simulink model "OMAP"  (R2018b)
settings: Solver=FixedStepDiscrete  StartTime=0.0  StopTime=10.0  FixedStep=0.01  RelTol=1e-3
values from neighbouring files (symbols this model uses):
  Clb_ICADirect_LaneDisp_StateFive = Simulink.Parameter    [omap_ver_442.m]
  Clb_ICADirect_LaneDisp_StateFour = Simulink.Parameter    [omap_ver_442.m]
  Clb_ICADirect_LaneDisp_StateOne = Simulink.Parameter    [omap_ver_442.m]
  Clb_ICADirect_LaneDisp_StateThree = Simulink.Parameter    [omap_ver_442.m]
  Clb_ICADirect_LaneDisp_StateTwo = Simulink.Parameter    [omap_ver_442.m]
  Clb_ICADirect_LaneDisp_StateZero = Simulink.Parameter    [omap_ver_442.m]
  Clb_ICADirect_LaneDispSW = Simulink.Parameter    [omap_ver_442.m]
  Clb_ICADirect_TrnLghtsCom_Switch = Simulink.Parameter    [omap_ver_442.m]
  Clb_ICADirect_TrnLghtsCom_Value = Simulink.Parameter    [omap_ver_442.m]
  Clb_ICADirect_TrnLghtsCrtl_Inhb = Simulink.Parameter    [omap_ver_442.m]
  OMAP_ACCAEB_EMSESC_Decel = Simulink.Parameter    [omap_ver_442.m]
  OMAP_ACCFCW_IC_Decel = Simulink.Parameter    [omap_ver_442.m]
  OMAP_clb_ACC_RVVReqType = Simulink.Parameter    [omap_ver_442.m]
  OMAP_clb_ACC_RVVReqType_Switch = Simulink.Parameter    [omap_ver_442.m]
  OMAP_clb_ACCHeadwayDisplay = Simulink.Parameter    [omap_ver_442.m]
  OMAP_clb_ACCHeadwayDisplay_Switch = Simulink.Parameter    [omap_ver_442.m]
  OMAP_clb_ACCHeadwayIcon = Simulink.Parameter    [omap_ver_442.m]
  OMAP_clb_ACCHeadwayIcon_Switch = Simulink.Parameter    [omap_ver_442.m]
  OMAP_clb_ACCMessagePrompt = Simulink.Parameter    [omap_ver_442.m]
  OMAP_clb_ACCMessagePrompt_Switch = Simulink.Parameter    [omap_ver_442.m]
  OMAP_clb_ACCRequestEPB = Simulink.Parameter    [omap_ver_442.m]
  OMAP_clb_ACCRequestEPB_Switch = Simulink.Parameter    [omap_ver_442.m]
  OMAP_clb_ACCSetSpeed = Simulink.Parameter    [omap_ver_442.m]
  OMAP_clb_ACCSetSpeed_Switch = Simulink.Parameter    [omap_ver_442.m]
  OMAP_clb_ACCSetSpeedDis = Simulink.Parameter    [omap_ver_442.m]
  OMAP_clb_ACCSetSpeedDis_Switch = Simulink.Parameter    [omap_ver_442.m]
  OMAP_clb_ACCState = Simulink.Parameter    [omap_ver_442.m]
  OMAP_clb_ACCState_Switch = Simulink.Parameter    [omap_ver_442.m]
  OMAP_clb_ACCStatusIconDis = Simulink.Parameter    [omap_ver_442.m]
  OMAP_clb_ACCStatusIconDis_Switch = Simulink.Parameter    [omap_ver_442.m]
  OMAP_clb_ACCTorqueReq = Simulink.Parameter    [omap_ver_442.m]
  OMAP_clb_ACCTorqueReq_Switch = Simulink.Parameter    [omap_ver_442.m]
  OMAP_clb_ADAS_State = Simulink.Parameter    [omap_ver_442.m]
  OMAP_clb_ADAS_State_Switch = Simulink.Parameter    [omap_ver_442.m]
  OMAP_clb_AEBAlertReq = Simulink.Parameter    [omap_ver_442.m]
  OMAP_clb_AEBAlertReq_Switch = Simulink.Parameter    [omap_ver_442.m]
  OMAP_clb_AEBBrakingProg = Simulink.Parameter    [omap_ver_442.m]
  OMAP_clb_AEBBrakingProg_Switch = Simulink.Parameter    [omap_ver_442.m]
  OMAP_clb_AEBFaultStatus = Simulink.Parameter    [omap_ver_442.m]
  OMAP_clb_AEBFaultStatus_Switch = Simulink.Parameter    [omap_ver_442.m]
  OMAP_clb_AEBMassageDisp = Simulink.Parameter    [omap_ver_442.m]
  OMAP_clb_AEBMassageDisp_Switch = Simulink.Parameter    [omap_ver_442.m]
  OMAP_clb_AEBState = Simulink.Parameter    [omap_ver_442.m]
  OMAP_clb_AEBState_Switch = Simulink.Parameter    [omap_ver_442.m]
  OMAP_clb_AEBSwitchStatus = Simulink.Parameter    [omap_ver_442.m]
  OMAP_clb_AEBSwitchStatus_Switch = Simulink.Parameter    [omap_ver_442.m]
  OMAP_clb_BrakeRequest = Simulink.Parameter    [omap_ver_442.m]
  OMAP_clb_BrakeRequest_Switch = Simulink.Parameter    [omap_ver_442.m]
  OMAP_clb_DecelerationSet = Simulink.Parameter    [omap_ver_442.m]
  OMAP_clb_DecelerationSet_Switch = Simulink.Parameter    [omap_ver_442.m]
  OMAP_clb_DecelerationType = Simulink.Parameter    [omap_ver_442.m]
  OMAP_clb_DecelerationType_Switch = Simulink.Parameter    [omap_ver_442.m]
  OMAP_clb_DeclControlReq = Simulink.Parameter    [omap_ver_442.m]
  OMAP_clb_DeclControlReq_Switch = Simulink.Parameter    [omap_ver_442.m]
  OMAP_clb_DownorUpGearMinTime = Simulink.Parameter    [omap_ver_442.m]
  OMAP_clb_DownorUpGearMinTime_Switch = Simulink.Parameter    [omap_ver_442.m]
  OMAP_clb_ELKPopupMessage = Simulink.Parameter    [omap_ver_442.m]
  OMAP_clb_ELKPopupMessage_Switch = Simulink.Parameter    [omap_ver_442.m]
  OMAP_clb_ELKSts = Simulink.Parameter    [omap_ver_442.m]
  OMAP_clb_ELKSts_Switch = Simulink.Parameter    [omap_ver_442.m]
  OMAP_clb_ESAFaultSt = Simulink.Parameter    [omap_ver_442.m]
  OMAP_clb_ESAFaultSt_Switch = Simulink.Parameter    [omap_ver_442.m]
  OMAP_clb_ESARequest = Simulink.Parameter    [omap_ver_442.m]
  OMAP_clb_ESARequest_Switch = Simulink.Parameter    [omap_ver_442.m]
  OMAP_clb_ESAState = Simulink.Parameter    [omap_ver_442.m]
  OMAP_clb_ESAState_Switch = Simulink.Parameter    [omap_ver_442.m]
  OMAP_clb_ESATorqueReq = Simulink.Parameter    [omap_ver_442.m]
  OMAP_clb_ESATorqueReq_Switch = Simulink.Parameter    [omap_ver_442.m]
  OMAP_clb_ESCDriveOff = Simulink.Parameter    [omap_ver_442.m]
  OMAP_clb_ESCDriveOff_Switch = Simulink.Parameter    [omap_ver_442.m]
  OMAP_clb_ESCHoldReq = Simulink.Parameter    [omap_ver_442.m]
  OMAP_clb_ESCHoldReq_Switch = Simulink.Parameter    [omap_ver_442.m]
  OMAP_clb_Handsoffwarning = Simulink.Parameter    [omap_ver_442.m]
  OMAP_clb_Handsoffwarning_Switch = Simulink.Parameter    [omap_ver_442.m]
  OMAP_clb_HapticAlarmReq = Simulink.Parameter    [omap_ver_442.m]
  OMAP_clb_HapticAlarmReq_Switch = Simulink.Parameter    [omap_ver_442.m]
  OMAP_clb_HMIPopupMassage = Simulink.Parameter    [omap_ver_442.m]
  OMAP_clb_HMIPopupMassage_Switch = Simulink.Parameter    [omap_ver_442.m]
  OMAP_clb_HWAActionSts = Simulink.Parameter    [omap_ver_442.m]
  OMAP_clb_HWAActionSts_Switch = Simulink.Parameter    [omap_ver_442.m]
  OMAP_clb_HWAMode = Simulink.Parameter    [omap_ver_442.m]
  OMAP_clb_HWAMode_Switch = Simulink.Parameter    [omap_ver_442.m]
  OMAP_clb_HWATurnOnIdctr = Simulink.Parameter    [omap_ver_442.m]
  OMAP_clb_HWATurnOnIdctr_Switch = Simulink.Parameter    [omap_ver_442.m]
  OMAP_clb_ICAMassageDisp = Simulink.Parameter    [omap_ver_442.m]
  OMAP_clb_ICAMassageDisp_Switch = Simulink.Parameter    [omap_ver_442.m]
  OMAP_clb_ICAStatusIcon = Simulink.Parameter    [omap_ver_442.m]
  OMAP_clb_ICAStatusIcon_Switch = Simulink.Parameter    [omap_ver_442.m]
  OMAP_clb_ISLCDriverRemind = Simulink.Parameter    [omap_ver_442.m]
  OMAP_clb_ISLCDriverRemind_Switch = Simulink.Parameter    [omap_ver_442.m]
  OMAP_clb_ISLCState = Simulink.Parameter    [omap_ver_442.m]
  OMAP_clb_ISLCState_Switch = Simulink.Parameter    [omap_ver_442.m]
  OMAP_clb_JAFaultSt = Simulink.Parameter    [omap_ver_442.m]
  OMAP_clb_JAFaultSt_Switch = Simulink.Parameter    [omap_ver_442.m]
  OMAP_clb_LCAPopupMessage = Simulink.Parameter    [omap_ver_442.m]
  OMAP_clb_LCAPopupMessage_Switch = Simulink.Parameter    [omap_ver_442.m]
  OMAP_clb_LCAStatusDisplay = Simulink.Parameter    [omap_ver_442.m]
  OMAP_clb_LCAStatusDisplay_Switch = Simulink.Parameter    [omap_ver_442.m]
  OMAP_clb_LDWStatusDisplay = Simulink.Parameter    [omap_ver_442.m]
  OMAP_clb_LDWStatusDisplay_Switch = Simulink.Parameter    [omap_ver_442.m]
  OMAP_clb_LDWWarningSt = Simulink.Parameter    [omap_ver_442.m]
  OMAP_clb_LDWWarningSt_Switch = Simulink.Parameter    [omap_ver_442.m]
  OMAP_clb_LightControlValid = Simulink.Parameter    [omap_ver_442.m]
  OMAP_clb_LightControlValid_Switch = Simulink.Parameter    [omap_ver_442.m]
  OMAP_clb_LKAActivation = Simulink.Parameter    [omap_ver_442.m]
  OMAP_clb_LKAActivation_Switch = Simulink.Parameter    [omap_ver_442.m]
  OMAP_clb_LKAAngleReq = Simulink.Parameter    [omap_ver_442.m]
  OMAP_clb_LKAAngleReq_Switch = Simulink.Parameter    [omap_ver_442.m]
  OMAP_clb_LKAMode = Simulink.Parameter    [omap_ver_442.m]
  OMAP_clb_LKAMode_Switch = Simulink.Parameter    [omap_ver_442.m]
  OMAP_clb_LKAorELK_CoolTime = Simulink.Parameter    [omap_ver_442.m]
  OMAP_clb_LKAState = Simulink.Parameter    [omap_ver_442.m]
  OMAP_clb_LKAState_Switch = Simulink.Parameter    [omap_ver_442.m]
  OMAP_clb_LKAStatusDisplay = Simulink.Parameter    [omap_ver_442.m]
  OMAP_clb_LKAStatusDisplay_Switch = Simulink.Parameter    [omap_ver_442.m]
  OMAP_clb_LKASwitchState = Simulink.Parameter    [omap_ver_442.m]
  OMAP_clb_LKASwitchState_Switch = Simulink.Parameter    [omap_ver_442.m]
  OMAP_clb_LKATorqFactReq = Simulink.Parameter    [omap_ver_442.m]
  OMAP_clb_LKATorqFactReq_Switch = Simulink.Parameter    [omap_ver_442.m]
  OMAP_clb_PrefillRequest = Simulink.Parameter    [omap_ver_442.m]
  ... (+36 more)
libraries: simulink x184, canmsglib x2
(part 6 of 14)

== system OMAP/Runnable_OMAP_10ms_sys/OMAP_Module/JABS_Direct ==
  Input_JABS : Inport
  Input_FDMM : Inport  Port=2
  Bus Creator10 : BusCreator  Inputs=8
  Bus Creator20 : BusCreator  Inputs=36
  Bus Creator4 : BusCreator  Inputs=7
  Bus Creator9 : BusCreator  Inputs=13
  Bus Selector8 : BusSelector  OutputSignals=JABSve_d_DbJACWStatus_convert,JABSve_d_DbFunFARCSta_convert,JABSve_d_DbPrefillReq_convert,JABSve_d_DbHapticAlarm_convert,JABSve_d_DbESCDriveOff_convert,JABSve_d_DbESCHoldReq_convert,JABSve_g_DbDecSetpoint_convert,JABSve_d_DbMDDdecRequest_convert,JABSve_d_DbMDDdecType_convert,JABSve_d_DbBraking_progress_convert,JABSve_d_DbAlertReq_convert,JABSve_d_DbSwitchStatus_convert,JABSve_d_DbTips_convert,JABSve_d_DbFltStatus_convert
  Constant{,2..4,14,16,19} (7 alike) : Constant  Value=0  OutDataTypeStr=uint8
  Constant1 : Constant  Value=0  OutDataTypeStr=single
  Constant13 : Constant  Value=6.2  OutDataTypeStr=single
  Constant15 : Constant  Value=3  OutDataTypeStr=uint8
  Constant17 : Constant  Value=-4000  OutDataTypeStr=single
  Constant18 : Constant  Value=-4000  OutDataTypeStr=single
  Data Type Conversion{1..3,15..24,26..27} (15 alike) : DataTypeConversion  OutDataTypeStr=uint8
  Data Type Conversion14 : DataTypeConversion  OutDataTypeStr=single
  OMAPve_g_Coefficient_toregulate_EPSNum : Constant  Value=0  OutDataTypeStr=single
  OMAPve_g_Column_angle_setpoint3F2Num : Constant  Value=0  OutDataTypeStr=single
  OMAPve_y_ACC_DesiredHeadway_DisplayNum2 : Constant  Value=0  OutDataTypeStr=uint8
  OMAPve_y_ACC_DesiredHeadway_Icon_BasicNum2 : Constant  Value=0  OutDataTypeStr=uint8
  OMAPve_y_ACC_Desired_Set_SpeedNum2 : Constant  Value=0  OutDataTypeStr=uint8
  OMAPve_y_ACC_HMI_TgtDisp_FlagNum2 : Constant  Value=0  OutDataTypeStr=uint8
  OMAPve_y_ACC_Pop_Up_MessageNum2 : Constant  Value=0  OutDataTypeStr=uint8
  OMAPve_y_ACC_Set_Speed_DisplayNum2 : Constant  Value=0  OutDataTypeStr=uint8
  OMAPve_y_ACC_Vehicle_Icon_DisplayNum2 : Constant  Value=0  OutDataTypeStr=uint8
  OMAPve_y_ADAS_ACCRequestEPBNum : Constant  Value=0  OutDataTypeStr=uint8
  OMAPve_y_ADAS_ELKStsNum1 : Constant  Value=0  OutDataTypeStr=uint8
  OMAPve_y_ADAS_HWAActionSts : Constant  Value=0  OutDataTypeStr=uint8
  OMAPve_y_ADAS_HWAMode : Constant  Value=0  OutDataTypeStr=uint8
  OMAPve_y_ADAS_HWATurnOnIndicator : Constant  Value=0  OutDataTypeStr=uint8
  OMAPve_y_ADAS_ISLCDriverRemind1 : Constant  Value=0  OutDataTypeStr=uint8
  OMAPve_y_ADAS_ISLCState1 : Constant  Value=0  OutDataTypeStr=uint8
  OMAPve_y_ADAS_LightControlValid : Constant  Value=0  OutDataTypeStr=uint8
  OMAPve_y_ADAS_TurnLightsCommand2 : Constant  Value=0  OutDataTypeStr=uint8
  OMAPve_y_AEB_Fault_Status_2 : Constant  Value=0  OutDataTypeStr=uint8
  OMAPve_y_General_state_of_LKA_function3F2Num : Constant  Value=0  OutDataTypeStr=uint8
  OMAPve_y_HMI_Popup_StatusNum2 : Constant  Value=0  OutDataTypeStr=uint8
  OMAPve_y_Hands_off_warningNum2 : Constant  Value=0  OutDataTypeStr=uint8
  OMAPve_y_ICA_HMI_Txt_DispNum2 : Constant  Value=0  OutDataTypeStr=uint8
  OMAPve_y_LDW_FlagNum2 : Constant  Value=0  OutDataTypeStr=uint8
  OMAPve_y_LDW_Status_DisplayNum2 : Constant  Value=0  OutDataTypeStr=uint8
  OMAPve_y_LKA_Mode_from_CameraNum2 : Constant  Value=0  OutDataTypeStr=uint8
  OMAPve_y_LKA_Status_DisplayNum2 : Constant  Value=0  OutDataTypeStr=uint8
  OMAPve_y_LKA_Switch_StateNum2 : Constant  Value=0  OutDataTypeStr=uint8
  OMAPve_y_LKA_action_indicationNum2 : Constant  Value=0  OutDataTypeStr=uint8
  OMAPve_y_Permit_to_know_if_LKA_or_LPA3F2Num : Constant  Value=0  OutDataTypeStr=uint8
  OMAPve_y_Power_steering_power_cut3F2Num : Constant  Value=0  OutDataTypeStr=uint8
  OMAPve_y_RVVACC_Vehiclespeed_request_typeNum2 : Constant  Value=0  OutDataTypeStr=uint8
  OMAPve_y_TARGET_POSITIONNum2 : Constant  Value=6  OutDataTypeStr=uint8
  OMAPve_y_TJA_status_iconNum2 : Constant  Value=0  OutDataTypeStr=uint8
  OMAPve_y_TSR_Vision_Only_Sign_TypeNum2 : Constant  Value=0  OutDataTypeStr=uint8
  OMAPve_y_Vehicle_Lane_DisplayNum2 : Constant  Value=0  OutDataTypeStr=uint8
  Terminator : Terminator
  JA_EMS : Outport
  JA_ESC : Outport  Port=2
  JA_EPS : Outport  Port=3
  JA_IC : Outport  Port=4
  JA_Input : Outport  Port=5
  wires:
  Bus Creator20/1 -> JA_IC/1  "JA_IC"
  Bus Selector8/12 -> Data Type Conversion26/1  "<JABSve_d_DbSwitchStatus_convert>"
  Bus Selector8/13 -> Data Type Conversion27/1  "<JABSve_d_DbTips_convert>"
  Bus Selector8/9 -> Data Type Conversion17/1  "<JABSve_d_DbMDDdecType_convert>"
  Data Type Conversion27/1 -> Bus Creator20/19  "OMAPve_y_AEB_tips_2"
  OMAPve_y_ICA_HMI_Txt_DispNum2/1 -> Bus Creator20/35  "OMAPve_y_ICA_HMI_Txt_Disp_2"
  OMAPve_y_TARGET_POSITIONNum2/1 -> Bus Creator20/22  "OMAPve_y_TARGET_POSITION_2"
  OMAPve_y_ACC_Vehicle_Icon_DisplayNum2/1 -> Bus Creator20/13  "OMAPve_y_ACC_Vehicle_Icon_Display_2"
  Bus Selector8/4 -> Data Type Conversion23/1  "<JABSve_d_DbHapticAlarm_convert>"
  OMAPve_y_HMI_Popup_StatusNum2/1 -> Bus Creator20/26  "OMAPve_y_HMI_Popup_Status_2"
  OMAPve_y_LKA_Status_DisplayNum2/1 -> Bus Creator20/31  "OMAPve_y_LKA_Status_Display_2"
  OMAPve_y_ACC_DesiredHeadway_DisplayNum2/1 -> Bus Creator20/9  "OMAPve_y_ACC_DesiredHeadway_Display_2"
  OMAPve_y_AEB_Fault_Status_2/1 -> Bus Creator20/17  "OMAPve_y_AEB_Fault_Status_2"
  Data Type Conversion24/1 -> Bus Creator20/16  "OMAPve_y_AEB_Alert_Req_2"
  OMAPve_y_ACC_HMI_TgtDisp_FlagNum2/1 -> Bus Creator20/21  "OMAPve_y_ACC_HMI_TgtDisp_Flag_2"
  Input_JABS/1 -> JA_Input/1, Bus Selector8/1
  OMAPve_y_LKA_Mode_from_CameraNum2/1 -> Bus Creator20/30  "OMAPve_y_LKA_Mode_from_Camera_2"
  Bus Selector8/11 -> Data Type Conversion24/1  "<JABSve_d_DbAlertReq_convert>"
  OMAPve_y_Vehicle_Lane_DisplayNum2/1 -> Bus Creator20/27  "OMAPve_y_Vehicle_Lane_Display_2"
  OMAPve_y_LKA_action_indicationNum2/1 -> Bus Creator20/33  "OMAPve_y_LKA_action_indication_2"
  Bus Selector8/1 -> Data Type Conversion22/1  "<JABSve_d_DbJACWStatus_convert>"
  Data Type Conversion15/1 -> Bus Creator9/9  "OMAPve_y_MDD_Decelerationcontrol_request_1"
  OMAPve_y_ACC_Desired_Set_SpeedNum2/1 -> Bus Creator20/11  "OMAPve_y_ACC_Desired_Set_Speed_2"
  OMAPve_y_TSR_Vision_Only_Sign_TypeNum2/1 -> Bus Creator20/8  "OMAPve_y_TSR_Vision_Only_Sign_Type_2"
  Constant15/1 -> Bus Creator4/7  "OMAPve_y_Function_Acc_status_1"
  Bus Creator4/1 -> JA_EMS/1  "JA_EMS"
  Constant13/1 -> Bus Creator4/5  "OMAPve_g_TminUp_or_downGear_1"
  OMAPve_y_LDW_Status_DisplayNum2/1 -> Bus Creator20/29  "OMAPve_y_LDW_Status_Display_2"
  Data Type Conversion26/1 -> Bus Creator20/18  "OMAPve_y_AEB_Switch_Status_2"
  Data Type Conversion22/1 -> Bus Creator9/1  "OMAPve_y_FCW_Status_1"
  Data Type Conversion17/1 -> Bus Creator9/10  "OMAPve_y_MDD_deceleration_type_1"
  Data Type Conversion14/1 -> Bus Creator9/8  "OMAPve_g_Deceleration_setpoint_device_1"
  Bus Selector8/3 -> Data Type Conversion16/1  "<JABSve_d_DbPrefillReq_convert>"
  Constant14/1 -> Bus Creator4/6  "OMAPve_y_stAcvTqWhlPTPotReq_1"
  Bus Selector8/8 -> Data Type Conversion20/1, Data Type Conversion15/1, Data Type Conversion21/1  "<JABSve_d_DbMDDdecRequest_convert>"
  Bus Creator9/1 -> JA_ESC/1  "JA_ESC"
  Constant16/1 -> Bus Creator4/1  "OMAPve_y_ACC_Engine_Start_Request_1"
  OMAPve_y_LKA_Switch_StateNum2/1 -> Bus Creator20/32  "OMAPve_y_LKA_Switch_State_2"
  OMAPve_y_ACC_DesiredHeadway_Icon_BasicNum2/1 -> Bus Creator20/10  "OMAPve_y_ACC_DesiredHeadway_Icon_Basic_2"
  OMAPve_y_LDW_FlagNum2/1 -> Bus Creator20/28  "OMAPve_y_LDW_Flag_2"
  Data Type Conversion16/1 -> Bus Creator9/4  "OMAPve_y_Prefill_request_1"
  Data Type Conversion18/1 -> Bus Creator9/2  "OMAPve_y_State_of_the_functionFARC_det_1"
  Constant19/1 -> Bus Creator4/4  "OMAPve_y_Powertrain_torquewheel_request_1"
  Data Type Conversion23/1 -> Bus Creator9/5  "OMAPve_y_Haptic_Alarm_1"
  Data Type Conversion19/1 -> Bus Creator9/3  "OMAPve_y_AEB_Status_1"
  OMAPve_y_RVVACC_Vehiclespeed_request_typeNum2/1 -> Bus Creator20/14  "OMAPve_y_RVVACC_Vehiclespeed_request_type_2"
  Bus Selector8/7 -> Data Type Conversion14/1  "<JABSve_g_DbDecSetpoint_convert>"
  Constant18/1 -> Bus Creator4/3  "OMAPve_g_ACCTqReq_1"
  OMAPve_y_Hands_off_warningNum2/1 -> Bus Creator20/25  "OMAPve_y_Hands_off_warning_2"
  OMAPve_y_TJA_status_iconNum2/1 -> Bus Creator20/36  "OMAPve_y_TJA_status_icon_2"
  Constant17/1 -> Bus Creator4/2  "OMAPve_g_PotACCTqReq_1"
  OMAPve_y_ACC_Pop_Up_MessageNum2/1 -> Bus Creator20/15  "OMAPve_y_ACC_Pop_Up_Message_2"
  Bus Selector8/2 -> Data Type Conversion19/1, Data Type Conversion18/1  "<JABSve_d_DbFunFARCSta_convert>"
  Data Type Conversion20/1 -> Bus Creator9/11  "OMAPve_y_Decel_Request_1"
  OMAPve_y_ACC_Set_Speed_DisplayNum2/1 -> Bus Creator20/12  "OMAPve_y_ACC_Set_Speed_Display_2"
  Data Type Conversion21/1 -> Bus Creator9/12  "OMAPve_y_AEB_Braking_progress_1"
  OMAPve_y_Power_steering_power_cut3F2Num/1 -> Bus Creator10/1  "OMAPve_y_Power_steering_power_cut3F2_2"
  Bus Creator10/1 -> JA_EPS/1  "JA_EPS"
  OMAPve_y_Permit_to_know_if_LKA_or_LPA3F2Num/1 -> Bus Creator10/5  "OMAPve_y_Permit_to_know_if_LKA_or_LPA3F2_2"
  OMAPve_g_Coefficient_toregulate_EPSNum/1 -> Bus Creator10/3  "OMAPve_g_Coefficient_toregulate_EPS_2"
  OMAPve_y_General_state_of_LKA_function3F2Num/1 -> Bus Creator10/2  "OMAPve_y_General_state_of_LKA_function3F2_2"
  OMAPve_g_Column_angle_setpoint3F2Num/1 -> Bus Creator10/4  "OMAPve_g_Column_angle_setpoint3F2_2"
  Input_FDMM/1 -> Terminator/1
  OMAPve_y_ADAS_ELKStsNum1/1 -> Bus Creator20/34  "OMAPve_y_ADAS_ELKSts_2"
  Data Type Conversion2/1 -> Bus Creator9/7  "OMAPve_y_ADAS_ESCHoldReq"
  Data Type Conversion1/1 -> Bus Creator9/6  "OMAPve_y_ADAS_ESCDriveOff"
  OMAPve_y_ADAS_ACCRequestEPBNum/1 -> Bus Creator9/13  "OMAPve_y_ADAS_ACCRequestEPB"
  Bus Selector8/5 -> Data Type Conversion1/1  "<JABSve_d_DbESCDriveOff_convert>"
  Bus Selector8/6 -> Data Type Conversion2/1  "<JABSve_d_DbESCHoldReq_convert>"
  Bus Selector8/10 -> ?  "<JABSve_d_DbBraking_progress_convert>"
  Data Type Conversion3/1 -> Bus Creator20/20  "OMAPve_y_ADAS_JAFaultSt_2"
  Bus Selector8/14 -> Data Type Conversion3/1  "<JABSve_d_DbFltStatus_convert>"
  OMAPve_y_ADAS_ISLCState1/1 -> Bus Creator20/23  "OMAPve_y_ADAS_ISLCState_2"
  OMAPve_y_ADAS_ISLCDriverRemind1/1 -> Bus Creator20/24  "OMAPve_y_ADAS_ISLCDriverRemind_2"
  OMAPve_y_ADAS_LightControlValid/1 -> Bus Creator20/6  "OMAPve_y_ADAS_LightControlValid_2"
  OMAPve_y_ADAS_HWAActionSts/1 -> Bus Creator20/4  "OMAPve_y_ADAS_HWAActionSts_2"
  OMAPve_y_ADAS_HWATurnOnIndicator/1 -> Bus Creator20/3  "OMAPve_y_ADAS_HWATurnOnIndicator_2"
  OMAPve_y_ADAS_HWAMode/1 -> Bus Creator20/7  "OMAPve_y_ADAS_HWAMode_2"
  OMAPve_y_ADAS_TurnLightsCommand2/1 -> Bus Creator20/5  "OMAPve_y_ADAS_TurnLightsCommand_2"
  Constant1/1 -> Bus Creator10/7  "OMAPve_g_ADAS_ESATorqueReq_2"
  Constant/1 -> Bus Creator10/6  "OMAPve_y_ADAS_ESAState_2"
  Constant2/1 -> Bus Creator10/8  "OMAPve_y_ADAS_ESARequest_2"
  Constant3/1 -> Bus Creator20/2  "OMAPve_y_ADAS_ESAFaultSt_2"
  Constant4/1 -> Bus Creator20/1  "OMAPve_y_ADAS_ELKPopupMessage_2"

== system OMAP/Runnable_OMAP_10ms_sys/OMAP_Module/LKAS_Direct ==
  Input_LKAS : Inport
  Input_FDMM : Inport  Port=2
  Bus Creator : BusCreator  Inputs=7
  Bus Creator1 : BusCreator  Inputs=36
  Bus Creator12 : BusCreator  Inputs=8
  Bus Creator5 : BusCreator  Inputs=13
  Bus Selector : BusSelector  OutputSignals=FDMMve_d_LkaFcnConf_convert
  Bus Selector9 : BusSelector  OutputSignals=LKASve_y_EPS_State_Control_convert,LKASve_g_EPS_Factor_Control_convert,LKASve_g_LKA_SWA_Control_convert,LKASve_y_EPS_LKA_Control_convert,LKASve_y_Hands_Off_Warning_convert,LKASve_y_HMI_Popup_Status_convert,LKASve_y_Vehicle_Lane_Display_convert,LKASve_y_LDW_Flag_convert,LKASve_y_LDW_Status_Display_convert,LKASve_y_LKA_Status_Display_convert,LKASve_y_LKA_Action_Indication_convert
  Constant{,2..3,5,21..22} (6 alike) : Constant  Value=0  OutDataTypeStr=uint8
  Constant1 : Constant  Value=0  OutDataTypeStr=single
  Data Type Conversion{28,31..39} (10 alike) : DataTypeConversion  OutDataTypeStr=uint8
  Data Type Conversion29 : DataTypeConversion  OutDataTypeStr=single
  Data Type Conversion30 : DataTypeConversion  OutDataTypeStr=single
  OMAPve_g_ACCTqReqNum : Constant  Value=-4000  OutDataTypeStr=single
  OMAPve_g_Deceleration_setpoint_deviceNum : Constant  Value=2.05  OutDataTypeStr=single
  OMAPve_g_PotACCTqReqNum : Constant  Value=-4000  OutDataTypeStr=single
  OMAPve_g_TminUp_or_downGearNum : Constant  Value=6.2  OutDataTypeStr=single
  OMAPve_y_ACC_DesiredHeadway_DisplayNum3 : Constant  Value=0  OutDataTypeStr=uint8
  OMAPve_y_ACC_DesiredHeadway_Icon_BasicNum3 : Constant  Value=0  OutDataTypeStr=uint8
  OMAPve_y_ACC_Desired_Set_SpeedNum3 : Constant  Value=0  OutDataTypeStr=uint8
  OMAPve_y_ACC_Engine_Start_RequestNum : Constant  Value=0  OutDataTypeStr=uint8
  OMAPve_y_ACC_HMI_TgtDisp_FlagNum3 : Constant  Value=0  OutDataTypeStr=uint8
  OMAPve_y_ACC_Pop_Up_MessageNum3 : Constant  Value=0  OutDataTypeStr=uint8
  OMAPve_y_ACC_Set_Speed_DisplayNum3 : Constant  Value=0  OutDataTypeStr=uint8
  OMAPve_y_ACC_Vehicle_Icon_DisplayNum3 : Constant  Value=0  OutDataTypeStr=uint8
  OMAPve_y_ADAS_ACCRequestEPBNum : Constant  Value=0  OutDataTypeStr=uint8
  OMAPve_y_ADAS_ELKStsNum1 : Constant  Value=0  OutDataTypeStr=uint8
  OMAPve_y_ADAS_ESCDriveOffNum : Constant  Value=0  OutDataTypeStr=uint8
  OMAPve_y_ADAS_ESCHoldReqNum : Constant  Value=0  OutDataTypeStr=uint8
  OMAPve_y_ADAS_HWAActionSts : Constant  Value=0  OutDataTypeStr=uint8
  OMAPve_y_ADAS_HWAMode : Constant  Value=0  OutDataTypeStr=uint8
  OMAPve_y_ADAS_HWATurnOnIndicator : Constant  Value=0  OutDataTypeStr=uint8
  OMAPve_y_ADAS_ISLCDriverRemind1 : Constant  Value=0  OutDataTypeStr=uint8
  OMAPve_y_ADAS_ISLCState1 : Constant  Value=0  OutDataTypeStr=uint8
  OMAPve_y_ADAS_JAFaultSt_2 : Constant  Value=0  OutDataTypeStr=uint8
  OMAPve_y_ADAS_LightControlValid : Constant  Value=0  OutDataTypeStr=uint8
  OMAPve_y_ADAS_TurnLightsCommand1 : Constant  Value=0  OutDataTypeStr=uint8
  OMAPve_y_AEB_Alert_ReqNum1 : Constant  Value=0  OutDataTypeStr=uint8
  OMAPve_y_AEB_Braking_progressNum : Constant  Value=0  OutDataTypeStr=uint8
  OMAPve_y_AEB_Fault_StatusNum1 : Constant  Value=0  OutDataTypeStr=uint8
  OMAPve_y_AEB_StatusNum : Constant  Value=0  OutDataTypeStr=uint8
  OMAPve_y_AEB_Switch_StatusNum1 : Constant  Value=0  OutDataTypeStr=uint8
  OMAPve_y_AEB_tipsNum1 : Constant  Value=0  OutDataTypeStr=uint8
  OMAPve_y_Decel_RequestNum : Constant  Value=0  OutDataTypeStr=uint8
  OMAPve_y_FCW_StatusNum : Constant  Value=10  OutDataTypeStr=uint8
  OMAPve_y_Function_Acc_statusNum : Constant  Value=3  OutDataTypeStr=uint8
  OMAPve_y_Haptic_AlarmNum : Constant  Value=0  OutDataTypeStr=uint8
  OMAPve_y_ICA_HMI_Txt_DispNum3 : Constant  Value=0  OutDataTypeStr=uint8
  OMAPve_y_MDD_Decelerationcontrol_requestNum : Constant  Value=0  OutDataTypeStr=uint8
  OMAPve_y_MDD_deceleration_typeNum : Constant  Value=0  OutDataTypeStr=uint8
  OMAPve_y_Powertrain_torquewheel_requestNum : Constant  Value=0  OutDataTypeStr=uint8
  OMAPve_y_Prefill_requestNum : Constant  Value=0  OutDataTypeStr=uint8
  OMAPve_y_RVVACC_Vehiclespeed_request_typeNum3 : Constant  Value=0  OutDataTypeStr=uint8
  OMAPve_y_State_of_the_functionFARC_detNum : Constant  Value=0  OutDataTypeStr=uint8
  OMAPve_y_TARGET_POSITIONNum3 : Constant  Value=6  OutDataTypeStr=uint8
  OMAPve_y_TJA_status_iconNum3 : Constant  Value=0  OutDataTypeStr=uint8
  OMAPve_y_TSR_Vision_Only_Sign_TypeNum3 : Constant  Value=0  OutDataTypeStr=uint8
  OMAPve_y_stAcvTqWhlPTPotReqNum : Constant  Value=0  OutDataTypeStr=uint8
  LKA_EMS : Outport
  LKA_ESC : Outport  Port=2
  LKA_EPS : Outport  Port=3
  LKA_IC : Outport  Port=4
  LKA_Input : Outport  Port=5
  wires:
  Bus Selector/1 -> Data Type Conversion39/1  "<FDMMve_d_LkaFcnConf_convert>"
  Bus Selector9/11 -> Data Type Conversion38/1  "<LKASve_y_LKA_Action_Indication_convert>"
  Bus Selector9/4 -> Data Type Conversion31/1  "<LKASve_y_EPS_LKA_Control_convert>"
  OMAPve_y_TSR_Vision_Only_Sign_TypeNum3/1 -> Bus Creator1/8  "OMAPve_y_TSR_Vision_Only_Sign_Type_2"
  Bus Selector9/5 -> Data Type Conversion32/1  "<LKASve_y_Hands_Off_Warning_convert>"
  Data Type Conversion39/1 -> Bus Creator1/32  "OMAPve_y_LKA_Switch_State_2"
  Data Type Conversion34/1 -> Bus Creator1/27  "OMAPve_y_Vehicle_Lane_Display_2"
  Bus Selector9/10 -> Data Type Conversion37/1  "<LKASve_y_LKA_Status_Display_convert>"
  Bus Creator12/1 -> LKA_EPS/1  "LKA_EPS"
  Bus Selector9/6 -> Data Type Conversion33/1  "<LKASve_y_HMI_Popup_Status_convert>"
  Data Type Conversion32/1 -> Bus Creator1/25  "OMAPve_y_Hands_off_warning_2"
  Input_FDMM/1 -> Bus Selector/1
  Constant22/1 -> Bus Creator1/30  "OMAPve_y_LKA_Mode_from_Camera_2"
  Constant21/1 -> Bus Creator12/1  "OMAPve_y_Power_steering_power_cut3F2_2"
  OMAPve_y_TJA_status_iconNum3/1 -> Bus Creator1/36  "OMAPve_y_TJA_status_icon_2"
  Data Type Conversion29/1 -> Bus Creator12/3  "OMAPve_g_Coefficient_toregulate_EPS_2"
  Input_LKAS/1 -> LKA_Input/1, Bus Selector9/1
  OMAPve_y_ACC_DesiredHeadway_DisplayNum3/1 -> Bus Creator1/9  "OMAPve_y_ACC_DesiredHeadway_Display_2"
  OMAPve_y_ACC_Pop_Up_MessageNum3/1 -> Bus Creator1/15  "OMAPve_y_ACC_Pop_Up_Message_2"
  OMAPve_y_ACC_Vehicle_Icon_DisplayNum3/1 -> Bus Creator1/13  "OMAPve_y_ACC_Vehicle_Icon_Display_2"
  Bus Selector9/8 -> Data Type Conversion35/1  "<LKASve_y_LDW_Flag_convert>"
  OMAPve_y_ICA_HMI_Txt_DispNum3/1 -> Bus Creator1/35  "OMAPve_y_ICA_HMI_Txt_Disp_2"
  OMAPve_y_TARGET_POSITIONNum3/1 -> Bus Creator1/22  "OMAPve_y_TARGET_POSITION_2"
  Data Type Conversion37/1 -> Bus Creator1/31  "OMAPve_y_LKA_Status_Display_2"
  OMAPve_y_RVVACC_Vehiclespeed_request_typeNum3/1 -> Bus Creator1/14  "OMAPve_y_RVVACC_Vehiclespeed_request_type_2"
  Data Type Conversion36/1 -> Bus Creator1/29  "OMAPve_y_LDW_Status_Display_2"
  Data Type Conversion38/1 -> Bus Creator1/33  "OMAPve_y_LKA_action_indication_2"
  OMAPve_y_AEB_Switch_StatusNum1/1 -> Bus Creator1/18  "OMAPve_y_AEB_Switch_Status_2"
  Bus Selector9/2 -> Data Type Conversion29/1  "<LKASve_g_EPS_Factor_Control_convert>"
  Data Type Conversion33/1 -> Bus Creator1/26  "OMAPve_y_HMI_Popup_Status_2"
  OMAPve_y_AEB_Fault_StatusNum1/1 -> Bus Creator1/17  "OMAPve_y_AEB_Fault_Status_2"
  OMAPve_y_ACC_Set_Speed_DisplayNum3/1 -> Bus Creator1/12  "OMAPve_y_ACC_Set_Speed_Display_2"
  Bus Selector9/1 -> Data Type Conversion28/1  "<LKASve_y_EPS_State_Control_convert>"
  OMAPve_y_ACC_HMI_TgtDisp_FlagNum3/1 -> Bus Creator1/21  "OMAPve_y_ACC_HMI_TgtDisp_Flag_2"
  Data Type Conversion28/1 -> Bus Creator12/2  "OMAPve_y_General_state_of_LKA_function3F2_2"
  Bus Selector9/7 -> Data Type Conversion34/1  "<LKASve_y_Vehicle_Lane_Display_convert>"
  Data Type Conversion31/1 -> Bus Creator12/5  "OMAPve_y_Permit_to_know_if_LKA_or_LPA3F2_2"
  OMAPve_y_ACC_DesiredHeadway_Icon_BasicNum3/1 -> Bus Creator1/10  "OMAPve_y_ACC_DesiredHeadway_Icon_Basic_2"
  Data Type Conversion35/1 -> Bus Creator1/28  "OMAPve_y_LDW_Flag_2"
  OMAPve_y_ACC_Desired_Set_SpeedNum3/1 -> Bus Creator1/11  "OMAPve_y_ACC_Desired_Set_Speed_2"
  Data Type Conversion30/1 -> Bus Creator12/4  "OMAPve_g_Column_angle_setpoint3F2_2"
  Bus Selector9/3 -> Data Type Conversion30/1  "<LKASve_g_LKA_SWA_Control_convert>"
  Bus Selector9/9 -> Data Type Conversion36/1  "<LKASve_y_LDW_Status_Display_convert>"
  OMAPve_y_AEB_tipsNum1/1 -> Bus Creator1/19  "OMAPve_y_AEB_tips_2"
  OMAPve_y_AEB_Alert_ReqNum1/1 -> Bus Creator1/16  "OMAPve_y_AEB_Alert_Req_2"
  OMAPve_g_TminUp_or_downGearNum/1 -> Bus Creator/5  "OMAPve_g_TminUp_or_downGear_1"
  Bus Creator/1 -> LKA_EMS/1  "LKA_EMS"
  OMAPve_g_PotACCTqReqNum/1 -> Bus Creator/2  "OMAPve_g_PotACCTqReq_1"
  OMAPve_y_Powertrain_torquewheel_requestNum/1 -> Bus Creator/4  "OMAPve_y_Powertrain_torquewheel_request_1"
  OMAPve_g_ACCTqReqNum/1 -> Bus Creator/3  "OMAPve_g_ACCTqReq_1"
  OMAPve_y_ACC_Engine_Start_RequestNum/1 -> Bus Creator/1  "OMAPve_y_ACC_Engine_Start_Request_1"
  OMAPve_y_Function_Acc_statusNum/1 -> Bus Creator/7  "OMAPve_y_Function_Acc_status_1"
  OMAPve_y_stAcvTqWhlPTPotReqNum/1 -> Bus Creator/6  "OMAPve_y_stAcvTqWhlPTPotReq_1"
  OMAPve_y_MDD_deceleration_typeNum/1 -> Bus Creator5/10  "OMAPve_y_MDD_deceleration_type_1"
  OMAPve_y_MDD_Decelerationcontrol_requestNum/1 -> Bus Creator5/9  "OMAPve_y_MDD_Decelerationcontrol_request_1"
  OMAPve_y_Decel_RequestNum/1 -> Bus Creator5/11  "OMAPve_y_Decel_Request_1"
  OMAPve_y_Prefill_requestNum/1 -> Bus Creator5/4  "OMAPve_y_Prefill_request_1"
  OMAPve_g_Deceleration_setpoint_deviceNum/1 -> Bus Creator5/8  "OMAPve_g_Deceleration_setpoint_device_1"
  OMAPve_y_AEB_StatusNum/1 -> Bus Creator5/3  "OMAPve_y_AEB_Status_1"
  OMAPve_y_AEB_Braking_progressNum/1 -> Bus Creator5/12  "OMAPve_y_AEB_Braking_progress_1"
  OMAPve_y_FCW_StatusNum/1 -> Bus Creator5/1  "OMAPve_y_FCW_Status_1"
  OMAPve_y_State_of_the_functionFARC_detNum/1 -> Bus Creator5/2  "OMAPve_y_State_of_the_functionFARC_det_1"
  OMAPve_y_Haptic_AlarmNum/1 -> Bus Creator5/5  "OMAPve_y_Haptic_Alarm_1"
  Bus Creator5/1 -> LKA_ESC/1  "LKA_ESC"
  OMAPve_y_ADAS_ELKStsNum1/1 -> Bus Creator1/34  "OMAPve_y_ADAS_ELKSts_2"
  OMAPve_y_ADAS_ESCHoldReqNum/1 -> Bus Creator5/7  "OMAPve_y_ADAS_ESCHoldReq"
  OMAPve_y_ADAS_ESCDriveOffNum/1 -> Bus Creator5/6  "OMAPve_y_ADAS_ESCDriveOff"
  OMAPve_y_ADAS_ACCRequestEPBNum/1 -> Bus Creator5/13  "OMAPve_y_ADAS_ACCRequestEPB"
  OMAPve_y_ADAS_JAFaultSt_2/1 -> Bus Creator1/20  "OMAPve_y_ADAS_JAFaultSt_2"
  OMAPve_y_ADAS_ISLCState1/1 -> Bus Creator1/23  "OMAPve_y_ADAS_ISLCState_2"
  OMAPve_y_ADAS_ISLCDriverRemind1/1 -> Bus Creator1/24  "OMAPve_y_ADAS_ISLCDriverRemind_2"
  OMAPve_y_ADAS_LightControlValid/1 -> Bus Creator1/6  "OMAPve_y_ADAS_LightControlValid_2"
  OMAPve_y_ADAS_HWAActionSts/1 -> Bus Creator1/4  "OMAPve_y_ADAS_HWAActionSts_2"
  OMAPve_y_ADAS_HWATurnOnIndicator/1 -> Bus Creator1/3  "OMAPve_y_ADAS_HWATurnOnIndicator_2"
  OMAPve_y_ADAS_HWAMode/1 -> Bus Creator1/7  "OMAPve_y_ADAS_HWAMode_2"
  OMAPve_y_ADAS_TurnLightsCommand1/1 -> Bus Creator1/5  "OMAPve_y_ADAS_TurnLightsCommand_2"
  Constant1/1 -> Bus Creator12/7  "OMAPve_g_ADAS_ESATorqueReq_2"
  Constant/1 -> Bus Creator12/6  "OMAPve_y_ADAS_ESAState_2"
  Constant2/1 -> Bus Creator12/8  "OMAPve_y_ADAS_ESARequest_2"
  Constant3/1 -> Bus Creator1/2  "OMAPve_y_ADAS_ESAFaultSt_2"
  Constant5/1 -> Bus Creator1/1  "OMAPve_y_ADAS_ELKPopupMessage_2"
  Bus Creator1/1 -> LKA_IC/1  "LKA_IC"

== system OMAP/Runnable_OMAP_10ms_sys/OMAP_Module/OTHER_Default_Arbitration ==
  Bus Creator27 : BusCreator  Inputs=5
  Data Type Conversion72 : DataTypeConversion  OutDataTypeStr=uint8
  Delay : Delay
  NOT : Logic  Operator=NOT  IconShape=distinctive  AllPortsSameDT=off  OutDataTypeStr=boolean
  OMAPve_y_ABS_ESP_power_cut_request2Num1 : Constant  Value=0  OutDataTypeStr=uint8
  OMAPve_y_ASR_connection_dis_demand2Num1 : Constant  Value=0  OutDataTypeStr=uint8
  OMAPve_y_ECU_operating_phaseNum1 : Constant  Value=9  OutDataTypeStr=uint8
  OMAPve_y_Radar_StateNum1 : Constant  Value=2  OutDataTypeStr=uint8
  Arbitration : Outport
  wires:
  Bus Creator27/1 -> Arbitration/1  "Arbitration"
  Data Type Conversion72/1 -> Bus Creator27/3  "OMAPve_y_TYPE_RAPPORT_2"
  Delay/1 -> NOT/1
  OMAPve_y_ASR_connection_dis_demand2Num1/1 -> Bus Creator27/2  "OMAPve_y_ASR_connection_dis_demand2_2"
  OMAPve_y_ABS_ESP_power_cut_request2Num1/1 -> Bus Creator27/1  "OMAPve_y_ABS_ESP_power_cut_request2_2"
  OMAPve_y_ECU_operating_phaseNum1/1 -> Bus Creator27/4  "OMAPve_y_ECU_operating_phase_2"
  OMAPve_y_Radar_StateNum1/1 -> Bus Creator27/5  "OMAPve_y_Radar_State_2"
  NOT/1 -> Delay/1, Data Type Conversion72/1

== system OMAP/Runnable_OMAP_10ms_sys/OMAP_Module/Subsystem ==
  Input_ACCS : Inport
  Input_AEBS : Inport  Port=2
  Input_JABS : Inport  Port=3
  Input_LKAS : Inport  Port=4
  Input_ELKS : Inport  Port=5
  Input_ESAS : Inport  Port=6
  Input_ICA : Inport  Port=7
  Input_FDMM : Inport  Port=8
  Input_IMAP : Inport  Port=9
  EMS_Arbitration : Subsystem
  EPS_Default_Arbitration : Subsystem
  ESC_Arbitration : Subsystem
  IC_Arbitration : Subsystem
  Out1 : Outport
  Out2 : Outport  Port=2
  Out3 : Outport  Port=3
  Out4 : Outport  Port=4
  wires:
  Input_ELKS/1 -> IC_Arbitration/5(Input_ELKS), EPS_Default_Arbitration/4(Input_ELKS), ESC_Arbitration/4(Input_ELKS)
  Input_ICA/1 -> IC_Arbitration/7(Input_ICA), EPS_Default_Arbitration/6(Input_ICA)
  Input_JABS/1 -> IC_Arbitration/3(Input_JABS), EPS_Default_Arbitration/2(Input_JABS), ESC_Arbitration/3(Input_JABS), EMS_Arbitration/3(Input_JABS)
  Input_FDMM/1 -> IC_Arbitration/8(Input_FDMM), EPS_Default_Arbitration/7(Input_FDMM), EMS_Arbitration/4(Input_FDMM), ESC_Arbitration/5(Input_FDMM)
  Input_ACCS/1 -> IC_Arbitration/1(Input_ACCS), ESC_Arbitration/1(Input_ACCS), EMS_Arbitration/1(Input_ACCS)
  Input_AEBS/1 -> EMS_Arbitration/2(Input_AEBS), IC_Arbitration/2(Input_AEBS), EPS_Default_Arbitration/1(Input_AEBS), ESC_Arbitration/2(Input_AEBS)
  Input_LKAS/1 -> EPS_Default_Arbitration/3(Input_LKAS), IC_Arbitration/4(Input_LKAS)
  Input_ESAS/1 -> EPS_Default_Arbitration/5(Input_ESAS), IC_Arbitration/6(Input_ESAS)
  IC_Arbitration/1(Arbitration_IC) -> Out4/1
  Input_IMAP/1 -> IC_Arbitration/9(Input_IMAP), EPS_Default_Arbitration/8(Input_IMAP), EMS_Arbitration/5(Input_IMAP), ESC_Arbitration/6(Input_IMAP)
  EPS_Default_Arbitration/1(Arbitration_EPS) -> Out3/1
  EMS_Arbitration/1(Arbitration_EMS) -> Out1/1
  ESC_Arbitration/1(Arbitration_ESC) -> Out2/1

== system OMAP/Runnable_OMAP_10ms_sys/OMAP_Module/Subsystem1 ==
  In1 : Inport
  Constant : Constant  Value=6  OutDataTypeStr=uint8
  Constant1 : Constant  Value=0  OutDataTypeStr=uint8
  Index Vector1 : MultiPortSwitch  DataPortOrder=Specify indices  Inputs=11  DataPortIndices={6,0}  OutDataTypeStr=uint8
  Out1 : Outport
  wires:
  Index Vector1/1 -> Out1/1
  In1/1 -> Index Vector1/1
  Constant/1 -> Index Vector1/2
  Constant1/1 -> Index Vector1/3

== system OMAP/Runnable_OMAP_10ms_sys/OMAP_Module/Subsystem2 ==
  OMAPve_g_ACCTqReq_1 : Inport
  OMAPve_y_Powertrain_torquewheel_request_1 : Inport  Port=2
  OMAPve_g_TminUp_or_downGear_1 : Inport  Port=3
  OMAPve_y_Function_Acc_status_1 : Inport  Port=4
  Bus Selector5 : BusSelector  OutputSignals=OMAP_clb_ACCTorqueReq_Switch,OMAP_clb_TorqueActivReq_Switch,OMAP_clb_DownorUpGearMinTime_Switch,OMAP_clb_ACCState_Switch
  Constant : Constant  Value=OMAP_clb_ACCTorqueReq
  Constant1 : Constant  Value=OMAP_clb_TorqueActivReq
  Constant2 : Constant  Value=OMAP_clb_DownorUpGearMinTime
  Constant3 : Constant  Value=OMAP_clb_ACCState
  Switch{,1..3} (4 alike) : Switch  Criteria=u2 > Threshold
  Out1 : Outport
  Out2 : Outport  Port=2
  Out3 : Outport  Port=3
  Out4 : Outport  Port=4
  wires:
  Bus Selector5/2 -> Switch1/2  "<OMAP_clb_TorqueActivReq_Switch>"
  Switch2/1 -> Out3/1
  OMAPve_y_Function_Acc_status_1/1 -> Switch3/3
  OMAPve_g_TminUp_or_downGear_1/1 -> Switch2/3
  OMAPve_y_Powertrain_torquewheel_request_1/1 -> Switch1/3
  Bus Selector5/1 -> Switch/2  "<OMAP_clb_ACCTorqueReq_Switch>"
  [ClbBus] -> Bus Selector5/1
  Bus Selector5/3 -> Switch2/2  "<OMAP_clb_DownorUpGearMinTime_Switch>"
  Bus Selector5/4 -> Switch3/2  "<OMAP_clb_ACCState_Switch>"
  OMAPve_g_ACCTqReq_1/1 -> Switch/3
  Switch1/1 -> Out2/1
  Switch3/1 -> Out4/1
  Switch/1 -> Out1/1
  Constant/1 -> Switch/1  "OMAP_clb_ACCTorqueReq"
  Constant1/1 -> Switch1/1  "OMAP_clb_TorqueActivReq"
  Constant2/1 -> Switch2/1  "OMAP_clb_DownorUpGearMinTime"
  Constant3/1 -> Switch3/1  "OMAP_clb_ACCState"

== system OMAP/Runnable_OMAP_10ms_sys/OMAP_Module/Subsystem3 ==
  OMAPve_g_Deceleration_setpoint_device_1 : Inport
  OMAPve_y_MDD_Decelerationcontrol_request_1 : Inport  Port=2
  OMAPve_y_Prefill_request_1 : Inport  Port=3
  OMAPve_y_ADAS_ESCDriveOff : Inport  Port=4
  OMAPve_y_ADAS_ESCHoldReq : Inport  Port=5
  OMAPve_y_MDD_deceleration_type_1 : Inport  Port=6
  OMAPve_y_AEB_Status_1 : Inport  Port=7
  OMAPve_y_Decel_Request_1 : Inport  Port=8
  OMAPve_y_AEB_Braking_progress_1 : Inport  Port=9
  OMAPve_y_Haptic_Alarm_1 : Inport  Port=10
  OMAPve_y_ADAS_ACCRequestEPB : Inport  Port=11
  Bus Selector5 : BusSelector  OutputSignals=OMAP_clb_DecelerationSet_Switch,OMAP_clb_DeclControlReq_Switch,OMAP_clb_PrefillRequest_Switch,OMAP_clb_ESCDriveOff_Switch,OMAP_clb_ESCHoldReq_Switch,OMAP_clb_DecelerationType_Switch,OMAP_clb_AEBState_Switch,OMAP_clb_BrakeRequest_Switch,OMAP_clb_AEBBrakingProg_Switch,OMAP_clb_HapticAlarmReq_Switch,OMAP_clb_ACCRequestEPB_Switch
  Constant10 : Constant  Value=OMAP_clb_AEBState
  Constant11 : Constant  Value=OMAP_clb_BrakeRequest
  Constant12 : Constant  Value=OMAP_clb_AEBBrakingProg
  Constant13 : Constant  Value=OMAP_clb_HapticAlarmReq
  Constant14 : Constant  Value=OMAP_clb_ACCRequestEPB
  Constant4 : Constant  Value=OMAP_clb_DecelerationSet
  Constant5 : Constant  Value=OMAP_clb_DeclControlReq
  Constant6 : Constant  Value=OMAP_clb_PrefillRequest
  Constant7 : Constant  Value=OMAP_clb_ESCDriveOff
  Constant8 : Constant  Value=OMAP_clb_ESCHoldReq
  Constant9 : Constant  Value=OMAP_clb_DecelerationType
  Switch{,1..10} (11 alike) : Switch  Criteria=u2 > Threshold
  Out1 : Outport
  Out2 : Outport  Port=2
  Out3 : Outport  Port=3
  Out4 : Outport  Port=4
  Out5 : Outport  Port=5
  Out6 : Outport  Port=6
  Out7 : Outport  Port=7
  Out8 : Outport  Port=8
  Out9 : Outport  Port=9
  Out10 : Outport  Port=10
  Out11 : Outport  Port=11
  wires:
  Switch/1 -> Out1/1
  Switch3/1 -> Out4/1
  Switch1/1 -> Out2/1
  OMAPve_g_Deceleration_setpoint_device_1/1 -> Switch/3
  Bus Selector5/4 -> Switch3/2  "<OMAP_clb_ESCDriveOff_Switch>"
  Bus Selector5/3 -> Switch2/2  "<OMAP_clb_PrefillRequest_Switch>"
  [ClbBus] -> Bus Selector5/1
  Bus Selector5/1 -> Switch/2  "<OMAP_clb_DecelerationSet_Switch>"
  OMAPve_y_MDD_Decelerationcontrol_request_1/1 -> Switch1/3
  OMAPve_y_Prefill_request_1/1 -> Switch2/3
  OMAPve_y_ADAS_ESCDriveOff/1 -> Switch3/3
  Switch2/1 -> Out3/1
  Bus Selector5/2 -> Switch1/2  "<OMAP_clb_DeclControlReq_Switch>"
  OMAPve_y_ADAS_ESCHoldReq/1 -> Switch4/3
  Bus Selector5/5 -> Switch4/2  "<OMAP_clb_ESCHoldReq_Switch>"
  Switch4/1 -> Out5/1
  Bus Selector5/6 -> Switch5/2  "<OMAP_clb_DecelerationType_Switch>"
  OMAPve_y_MDD_deceleration_type_1/1 -> Switch5/3
  Switch5/1 -> Out6/1
  Bus Selector5/7 -> Switch6/2  "<OMAP_clb_AEBState_Switch>"
  OMAPve_y_AEB_Status_1/1 -> Switch6/3
  Switch6/1 -> Out7/1
  Bus Selector5/8 -> Switch7/2  "<OMAP_clb_BrakeRequest_Switch>"
  OMAPve_y_Decel_Request_1/1 -> Switch7/3
  Switch7/1 -> Out8/1
  Switch8/1 -> Out9/1
  Bus Selector5/9 -> Switch8/2  "<OMAP_clb_AEBBrakingProg_Switch>"
  OMAPve_y_AEB_Braking_progress_1/1 -> Switch8/3
  Bus Selector5/10 -> Switch9/2  "<OMAP_clb_HapticAlarmReq_Switch>"
  Switch9/1 -> Out10/1
  OMAPve_y_Haptic_Alarm_1/1 -> Switch9/3
  Bus Selector5/11 -> Switch10/2  "<OMAP_clb_ACCRequestEPB_Switch>"
  OMAPve_y_ADAS_ACCRequestEPB/1 -> Switch10/3
  Switch10/1 -> Out11/1
  Constant4/1 -> Switch/1  "OMAP_clb_DecelerationSet"
  Constant5/1 -> Switch1/1  "OMAP_clb_DeclControlReq"
  Constant6/1 -> Switch2/1  "OMAP_clb_PrefillRequest"
  Constant7/1 -> Switch3/1  "OMAP_clb_ESCDriveOff"
  Constant8/1 -> Switch4/1  "OMAP_clb_ESCHoldReq"
  Constant9/1 -> Switch5/1  "OMAP_clb_DecelerationType"
  Constant10/1 -> Switch6/1  "OMAP_clb_AEBState"
  Constant11/1 -> Switch7/1  "OMAP_clb_BrakeRequest"
  Constant12/1 -> Switch8/1  "OMAP_clb_AEBBrakingProg"
  Constant13/1 -> Switch9/1  "OMAP_clb_HapticAlarmReq"
  Constant14/1 -> Switch10/1  "OMAP_clb_ACCRequestEPB"

== system OMAP/Runnable_OMAP_10ms_sys/OMAP_Module/Subsystem4 ==
  OMAPve_y_General_state_of_LKA_function3F2_2 : Inport
  OMAPve_g_Coefficient_toregulate_EPS_2 : Inport  Port=2
  OMAPve_g_Column_angle_setpoint3F2_2 : Inport  Port=3
  OMAPve_y_Permit_to_know_if_LKA_or_LPA3F2_2 : Inport  Port=4
  OMAPve_y_ADAS_ESAState_2 : Inport  Port=5
  OMAPve_g_ADAS_ESATorqueReq_2 : Inport  Port=6
  OMAPve_y_ADAS_ESARequest_2 : Inport  Port=7
  Bus Selector5 : BusSelector  OutputSignals=OMAP_clb_LKAState_Switch,OMAP_clb_LKATorqFactReq_Switch,OMAP_clb_LKAAngleReq_Switch,OMAP_clb_LKAActivation_Switch,OMAP_clb_ESAState_Switch,OMAP_clb_ESATorqueReq_Switch,OMAP_clb_ESARequest_Switch
  Constant15 : Constant  Value=OMAP_clb_LKAState
  Constant16 : Constant  Value=OMAP_clb_LKATorqFactReq
  Constant17 : Constant  Value=OMAP_clb_LKAAngleReq
  Constant18 : Constant  Value=OMAP_clb_LKAActivation
  Constant19 : Constant  Value=OMAP_clb_ESAState
  Constant20 : Constant  Value=OMAP_clb_ESATorqueReq
  Constant21 : Constant  Value=OMAP_clb_ESARequest
  Switch{,1..6} (7 alike) : Switch  Criteria=u2 > Threshold
  Out1 : Outport
  Out2 : Outport  Port=2
  Out3 : Outport  Port=3
  Out4 : Outport  Port=4
  Out5 : Outport  Port=5
  Out6 : Outport  Port=6
  Out7 : Outport  Port=7
  wires:
  Switch/1 -> Out1/1
  Switch3/1 -> Out4/1
  Switch1/1 -> Out2/1
  OMAPve_y_General_state_of_LKA_function3F2_2/1 -> Switch/3
  Bus Selector5/4 -> Switch3/2  "<OMAP_clb_LKAActivation_Switch>"
  Bus Selector5/3 -> Switch2/2  "<OMAP_clb_LKAAngleReq_Switch>"
  [ClbBus] -> Bus Selector5/1
  Bus Selector5/1 -> Switch/2  "<OMAP_clb_LKAState_Switch>"
  OMAPve_g_Coefficient_toregulate_EPS_2/1 -> Switch1/3
  OMAPve_g_Column_angle_setpoint3F2_2/1 -> Switch2/3
  OMAPve_y_Permit_to_know_if_LKA_or_LPA3F2_2/1 -> Switch3/3
  Switch2/1 -> Out3/1
  Bus Selector5/2 -> Switch1/2  "<OMAP_clb_LKATorqFactReq_Switch>"
  Bus Selector5/5 -> Switch4/2  "<OMAP_clb_ESAState_Switch>"
  OMAPve_y_ADAS_ESAState_2/1 -> Switch4/3
  Switch4/1 -> Out5/1
  Bus Selector5/6 -> Switch5/2  "<OMAP_clb_ESATorqueReq_Switch>"
  OMAPve_g_ADAS_ESATorqueReq_2/1 -> Switch5/3
  Switch5/1 -> Out6/1
  Bus Selector5/7 -> Switch6/2  "<OMAP_clb_ESARequest_Switch>"
  OMAPve_y_ADAS_ESARequest_2/1 -> Switch6/3
  Switch6/1 -> Out7/1
  Constant15/1 -> Switch/1  "OMAP_clb_LKAState"
  Constant16/1 -> Switch1/1  "OMAP_clb_LKATorqFactReq"
  Constant17/1 -> Switch2/1  "OMAP_clb_LKAAngleReq"
  Constant18/1 -> Switch3/1  "OMAP_clb_LKAActivation"
  Constant19/1 -> Switch4/1  "OMAP_clb_ESAState"
  Constant20/1 -> Switch5/1  "OMAP_clb_ESATorqueReq"
  Constant21/1 -> Switch6/1  "OMAP_clb_ESARequest"
